simulink model "Q8"  (R2018b)
settings: Solver=VariableStepAuto  StartTime=0.0  StopTime=10.0  RelTol=1e-3
undefined symbols (not defined in the file): C, G, K, T
libraries: slctrlblks x1
settings Model: Creator=xpess  LastModifiedBy=xpess

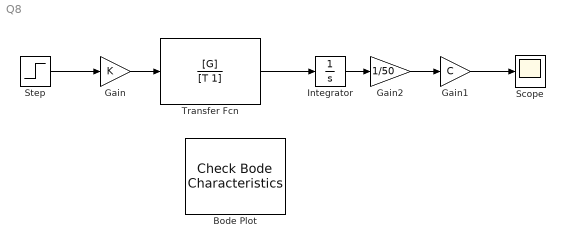
== system Q8 ==
  Bode Plot : slctrlblks/Model Verification/Check Bode  Characteristics  InstantiateOnLoad=on  SaveOperatingPoints=off  LinearizationIOs={'/Step', 1, 'in', 'on', '';'/Gain1', 1, 'out', 'on', ''}  LinearizeAt=SnapshotTimes  SnapshotTimes=[0]  TriggerType=rising  SampleTime=auto  RateConversionMethod=zoh  PreWarpFreq=10  UseExactDelayModel=off  UseFullBlockNameLabels=off  UseBusSignalLabels=off  enabled=on  stopWhenAssertionFail=off  export=off  ViewDlgPos=[641.666666666667 41.6666666666667 638.666666666667 599.333333333333]  OpenViewOnLoad=on  LaunchViewOnOpen=on  FrequencyUnits=rad/s  MagnitudeUnits=dB  PhaseUnits=deg  TimeUnits=seconds  EnableUpperBound=off  UpperBoundFrequencies=[]  UpperBoundMagnitudes=[]  EnableLowerBound=off  LowerBoundFrequencies=[]  LowerBoundMagnitudes=[]
      settings: SourceProductName=Simulink Control Design
  Gain : Gain  Gain=K
  Gain1 : Gain  Gain=C
  Gain2 : Gain  Gain=1/50
  Integrator : Integrator
  Scope : Scope
  Step : Step  Time=0  SampleTime=0
  Transfer Fcn : TransferFcn  Numerator=[G]  Denominator=[T 1]
  wires:
  Integrator/1 -> Gain2/1
  Transfer Fcn/1 -> Integrator/1
  Step/1 -> Gain/1
  Gain/1 -> Transfer Fcn/1
  Gain2/1 -> Gain1/1
  Gain1/1 -> Scope/1
